simulink model "maglev_2d"  (R2024b)
settings: Solver=VariableStepAuto  StartTime=0.0  StopTime=100  RelTol=1e-3
model workspace (MAT data in the model file):
  params.solenoids.x = [0.02 -0.02 0 0]
  params.solenoids.y = [0 0 0.02 -0.02]
  params.solenoids.r = [0.00925 0.00925 0.00925 0.00925]
  params.solenoids.l = [0.012 0.012 0.012 0.012]
  params.solenoids.z = [0.006 0.006 0.006 0.006]
  params.solenoids.nw = 480
  params.permanent.x = [0.028 -0.028 0.028 -0.028]
  params.permanent.y = [0.028 0.028 -0.028 -0.028]
  params.permanent.r = [0.01 0.01 0.01 0.01]
  params.permanent.l = [0.009 0.009 0.009 0.009]
  params.permanent.z = [0.0046 0.0046 0.0046 0.0046]
  params.permanent.J = 1.1
  params.magnet.r = 0.025
  params.magnet.l = 0.005
  params.magnet.J = -1
  params.magnet.m = 0.077
  params.magnet.I = [1.21916666667e-05 1.21916666667e-05 2.40625e-05]
  params.magnet.n = 100
  params.sensors.x = [0 -0.019 -0.019]
  params.sensors.y = [0 0.019 -0.019]
  params.sensors.z = [0 0 0]
  params.physical.g = 9.81
  params.physical.mu0 = 1.25663706144e-06
libraries: slpidlib x1
settings Model: ParameterArgumentNames=params  Creator=hansae  LastModifiedBy=morad
settings OptimizationCC: ReuseModelBlockBuffer=off
settings RTWCC: GPUComputeCapability=3.5

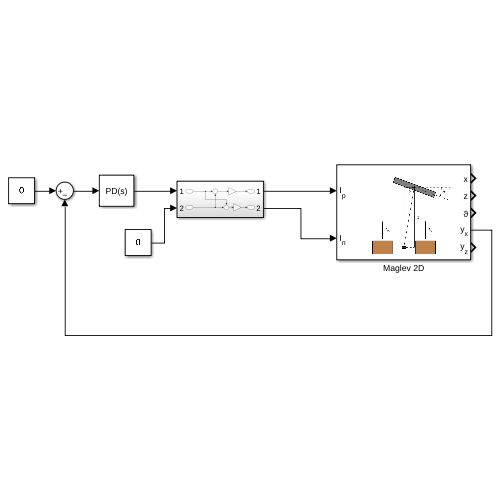
[thumbnail: Simulink's stored preview of the top-level diagram]
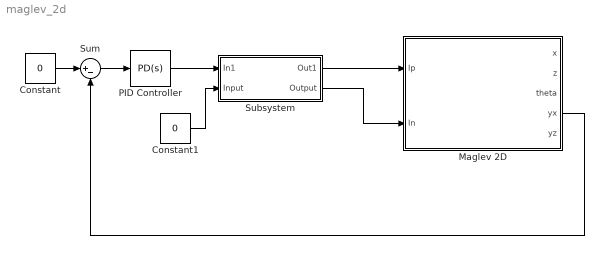
== system maglev_2d ==
  Constant : Constant  Value=0
  Constant1 : Constant  Value=0
  Maglev 2D : Subsystem
      mask Display:
      | image('$imagefile'); % Use "Edit Image" on toolstrip to change.
      | port_label('input', 1, 'I_p','interpreter','tex')
      | port_label('input', 2, 'I_n','interpreter','tex')
      | port_label('output', 1, 'x','interpreter','tex')
      | port_label('output', 2, 'z','interpreter','tex')
      | port_label('output', 3, '\vartheta','interpreter','tex')
      | port_label('output', 4, 'y_x','interpreter','tex')
      | port_label('output', 5, 'y_z','interpreter','tex')
  PID Controller : slpidlib/PID Controller  Controller=PD  Form=Parallel  TimeDomain=Continuous-time  UseExternalTs=off  SampleTime=-1  IntegratorMethod=Forward Euler  FilterMethod=Forward Euler  ControllerParametersSource=internal  P=5000  I=1  UseKiTs=off  D=100  UseExternalDerivativeSource=off  N=100  UseFilter=on  TunerSelectOption=Frequency Response Based  InitialConditionSource=internal  InitialConditionForIntegrator=0  InitialConditionForFilter=0  DifferentiatorICPrevScaledInput=0  ExternalReset=none  TrackingMode=off  Kt=1  LimitOutput=off  SatLimitsSource=internal  UpperSaturationLimit=inf  LowerSaturationLimit=-inf  LinearizeAsGain=on  AntiWindupMode=none  Kb=1  LimitIntegrator=off  UpperIntegratorSaturationLimit=inf  LowerIntegratorSaturationLimit=-inf  POutMin=[]  POutMax=[]  IOutMin=[]  IOutMax=[]  DOutMin=[]  DOutMax=[]  NOutMin=[]  NOutMax=[]  SumOutMin=[]  SumOutMax=[]  SaturationOutMin=[]  SaturationOutMax=[]  PParamMin=[]  PParamMax=[]  IParamMin=[]  IParamMax=[]  DParamMin=[]  DParamMax=[]  NParamMin=[]  NParamMax=[]  KbParamMin=[]  KbParamMax=[]  KtParamMin=[]  KtParamMax=[]  KbOutMin=[]  KbOutMax=[]  KtOutMin=[]  KtOutMax=[]  IntegratorOutMin=[]  IntegratorOutMax=[]  FilterOutMin=[]  FilterOutMax=[]  SumI1OutMin=[]  SumI1OutMax=[]  SumI2OutMin=[]  SumI2OutMax=[]  SumI3OutMin=[]  SumI3OutMax=[]  SumI4OutMin=[]  SumI4OutMax=[]  SumDOutMin=[]  SumDOutMax=[]  DifferentiatorOutMin=[]  DifferentiatorOutMax=[]  FilterDiffOutCoefMin=[]  FilterDiffOutCoefMax=[]  ReciprocalOutMin=[]  ReciprocalOutMax=[]  SumDenOutMin=[]  SumDenOutMax=[]  SumNumOutMin=[]  SumNumOutMax=[]  DivideOutMin=[]  DivideOutMax=[]  UdiffTsProdOutMin=[]  UdiffTsProdOutMax=[]  NTsProdOutMin=[]  NTsProdOutMax=[]  UintegralTsProdOutMin=[]  UintegralTsProdOutMax=[]  UngainTsProdOutMin=[]  UngainTsProdOutMax=[]  ClampingZeroOutDataTypeStr=Inherit: Inherit via back propagation  ClampingZeroOutMin=[]  ClampingZeroOutMax=[]  FilterDenConstantOutDataTypeStr=Inherit: Inherit via back propagation  FilterDenConstantOutMin=[]  FilterDenConstantOutMax=[]  PCopyOutDataTypeStr=Inherit: Inherit via back propagation  PCopyOutMin=[]  PCopyOutMax=[]  NCopyOutDataTypeStr=Inherit: Inherit via back propagation  NCopyOutMin=[]  NCopyOutMax=[]  IntegratorContinuousStateAttributes=''  IntegratorStateMustResolveToSignalObject=off  IntegratorRTWStateStorageClass=Auto  FilterContinuousStateAttributes=''  FilterStateMustResolveToSignalObject=off  FilterRTWStateStorageClass=Auto  ParallelPVariant=InternalParameters  IdealPVariant=Disabled  IVariant=Disabled  DVariant=InternalParameters  IntegratorVariant=Disabled  SatVariant=Disabled  AWVariant=Disabled  PCopyVariant=Disabled  TRVariant=Disabled  FdbkBlocksVariant=Forward  IdealPFdbkVariant=Disabled  SatFdbkVariant=Disabled  DerivativeFilterVariant=ContFilter  NVariant=InternalParameters  NCopyVariant=Disabled  FilterICVariant=InternalICsFilter  IntegratorICVariant=Disabled  ExternalResetVariant=Disabled  TRSumVariant=Passthrough  SumFdbkVariant=Disabled  SumVariant=Sum_PD  TsampFilterVariant=InternalTs  TsampNgainVariant=Passthrough  TsampIntegralVariant=Disabled_SignalSpec  ExternalSaturationOutDataTypeStr=Inherit: Same as second input  DerivativeSourceVariant=ErrorSignal  PreIntVariant=InternalPreInt
  Subsystem : Subsystem
  Sum : Sum  Inputs=|+-
  wires:
  Maglev 2D/4(yx) -> Sum/2
  Constant/1 -> Sum/1
  Sum/1 -> PID Controller/1
  PID Controller/1 -> Subsystem/1(In1)
  Constant1/1 -> Subsystem/2(Input)
  Subsystem/1(Out1) -> Maglev 2D/1(Ip)
  Subsystem/2(Output) -> Maglev 2D/2(In)

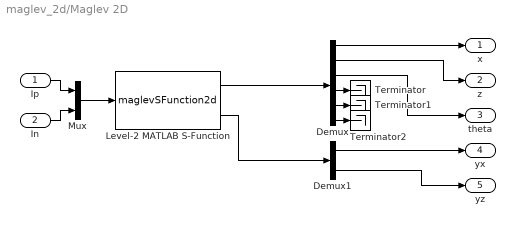
== system maglev_2d/Maglev 2D ==
  Ip : Inport
  In : Inport  Port=2
  Demux : Demux  Outputs=6
  Demux1 : Demux  Outputs=2
  Level-2 MATLAB S-Function : M-S-Function  FunctionName=maglevSFunction2d
  Mux : Mux  Inputs=2
  Terminator : Terminator
  Terminator1 : Terminator
  Terminator2 : Terminator
  x : Outport
  z : Outport  Port=2
  theta : Outport  Port=3
  yx : Outport  Port=4
  yz : Outport  Port=5
  wires:
  Demux/1 -> x/1
  Demux/3 -> theta/1
  Demux1/1 -> yx/1
  Demux1/2 -> yz/1
  Mux/1 -> Level-2 MATLAB S-Function/1
  Ip/1 -> Mux/1
  In/1 -> Mux/2
  Demux/4 -> Terminator/1
  Demux/5 -> Terminator1/1
  Demux/6 -> Terminator2/1
  Level-2 MATLAB S-Function/2 -> Demux1/1
  Level-2 MATLAB S-Function/1 -> Demux/1
  Demux/2 -> z/1

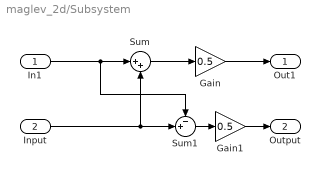
== system maglev_2d/Subsystem ==
  In1 : Inport
  Input : Inport  Port=2
  Gain : Gain  Gain=0.5
  Gain1 : Gain  Gain=0.5
  Sum : Sum  Inputs=|++
  Sum1 : Sum  Inputs=-+|
  Out1 : Outport
  Output : Outport  Port=2
  wires:
  In1/1 -> Sum1/1, Sum/1
  Sum/1 -> Gain/1
  Gain/1 -> Out1/1
  Input/1 -> Sum1/2, Sum/2
  Sum1/1 -> Gain1/1
  Gain1/1 -> Output/1
